simulink model "USRP_toFile"  (R2020a)
settings: Solver=FixedStepAuto  StartTime=0.0  StopTime=2  RelTol=1e-3
StartFcn:
  | tc = clock; %当前时间
  | time_str = sprintf('%d%02d%02d_%02d%02d%02d', tc(1),tc(2),tc(3),tc(4),tc(5),floor(tc(6)));
StopFcn:
  | system(['ren B210_data.dat B210_',time_str,'_ch1.dat'])
  | clearvars tc time_str
libraries: dspsnks4 x1, commsdrhw_v2 x1
settings Model: SimulationMode=rapid-accelerator  Creator=longt  LastModifiedBy=longt
settings DataIOCC: SaveOutput=off  SignalLogging=off  DSMLogging=off  SaveTime=off  ReturnWorkspaceOutputs=off

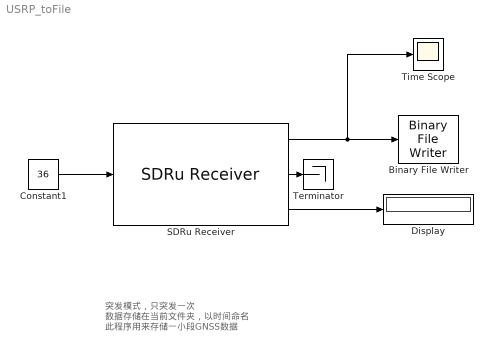
== system USRP_toFile ==
  note: 突发模式，只突发一次
      | 数据存储在当前文件夹，以时间命名
      | 此程序用来存储一小段GNSS数据
  Binary File Writer : dspsnks4/Binary File Writer  Filename=B210_data.dat  HeaderStructure=struct([])  SimulateUsing=Code generation
      settings: SourceProductBaseCode=DS
  Constant1 : Constant  Value=36
  Display : Display
  SDRu Receiver : commsdrhw_v2/SDRu Receiver  rxtx=rx  initializeIPAddress=0  devMap=10  USRP2_IP=192.168.10.2  USRP_IP_X300=192.168.10.2  USRP_IP_X310=No devices found  USRP_IP_N300=192.168.10.2  USRP_IP_N310=192.168.10.2  USRP_IP_N320=192.168.10.2  USRP_serialNumB200=No devices found  USRP_serialNumB210=315F337  platform=B210  prevPlatform=B210  lastIPAddressPopup=192.168.10.2  USRP_ID=315F337  LastIPAddress=192.168.10.2  IsTwinRXDaughterboard=off  EnableTwinRXPhaseSync=off  losrc=0  ChannelMapping=1  centerFrequencySrc=Dialog  centerFrequency=1575.42e6  loOffsetSrc=Dialog  loOffset=0  gainSrc=Input port  gain=32  PPSSource=Internal  clockSource=Internal  masterClkRateParam=16000000  masterClkRateB200=32e6  masterClkRateB210=16e6  masterClkRateX300=200e6  masterClkRateX310=200e6  masterClkRateN300=125e6  masterClkRateN310=125e6  masterClkRateN320=200e6  masterClkRate=100e6  masterClkRateTwinRX=200e6  decimInterpSrc=Dialog  decimInterpPort=512  lastDecimSource=Dialog  decimInterp=4  USRP2_IP_NUM=[51 49 53 70 51 51 55]  sampleRate=4000000  sampleTime=2.5e-07  TransportDataType=int16  overrunUnderrunPort=on  outputDatatype=Same as transport data type  frameLength=4000  HOST_DATA_PORT=0  HOST_CONTROL_PORT=0  USRP2_DATA_PORT=0  USRP2_CONTROL_PORT=0  bufferMode=Continuous streaming  EnableBurstMode=on  NumFramesInBurst=2000
      settings: SourceProductBaseCode=USRP
  Terminator : Terminator
  Time Scope : Scope
  wires:
  Constant1/1 -> SDRu Receiver/1
  SDRu Receiver/2 -> Terminator/1
  SDRu Receiver/1 -> Time Scope/1, Binary File Writer/1
  SDRu Receiver/3 -> Display/1
